simulink model "testsim_1"  (R2017b)
settings: Solver=VariableStepAuto  StartTime=0.0  StopTime=10.0  RelTol=1e-3
undefined symbols (not defined in the file or in its folder): a1, a2, a3
settings Model: Creator=rishi  LastModifiedBy=rishi

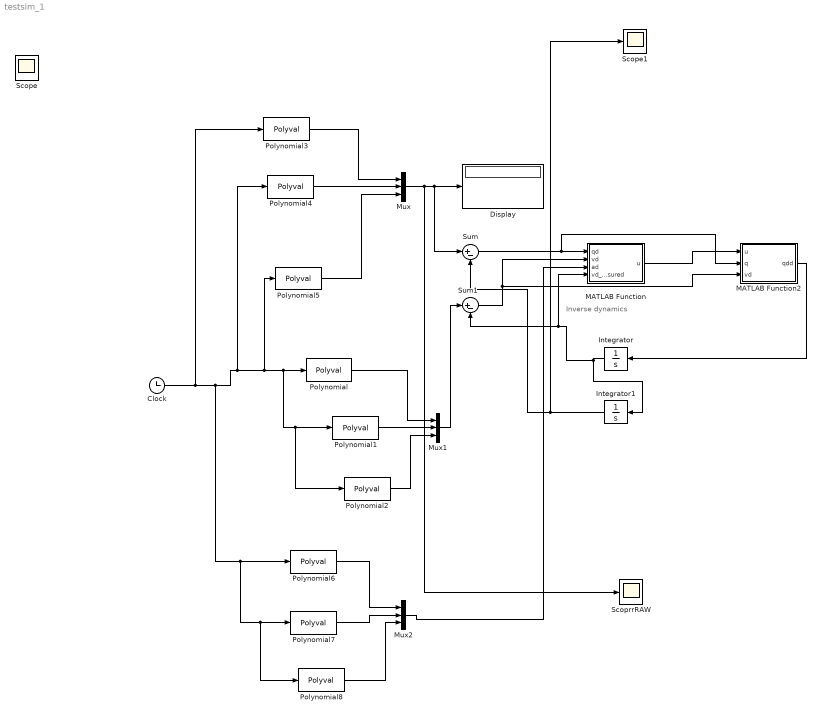
== system testsim_1 ==
  note: Inverse dynamics
  Clock : Clock
  Display : Display
  Integrator : Integrator
  Integrator1 : Integrator
  MATLAB Function : MATLAB Function  TreatAsAtomicUnit=on
  MATLAB Function2 : MATLAB Function  TreatAsAtomicUnit=on
  Mux : Mux  Inputs=3
  Mux1 : Mux  Inputs=3
  Mux2 : Mux  Inputs=3
  Polynomial : Polyval  Coefs=[a1(2) 2*a1(3) 3*a1(4)]
  Polynomial1 : Polyval  Coefs=[a2(2) 2*a2(3) 3*a2(4)]
  Polynomial2 : Polyval  Coefs=[a3(2) 2*a3(3) 3*a3(4)]
  Polynomial3 : Polyval  Coefs=[ a1(1) a1(2) a1(3) a1(4)]
  Polynomial4 : Polyval  Coefs=[ a2(1) a2(2) a2(3) a2(4)]
  Polynomial5 : Polyval  Coefs=[ a3(1) a3(2) a3(3) a3(4)]
  Polynomial6 : Polyval  Coefs=[2*a1(3) 6*a1(4)]
  Polynomial7 : Polyval  Coefs=[2*a2(3) 6*a2(4)]
  Polynomial8 : Polyval  Coefs=[2*a3(3) 6*a3(4)]
  Scope1 : Scope
  "ScoprrRAW " : Scope
  Sum : Sum  Inputs=|+-
  Sum1 : Sum  Inputs=|+-
  Scope : Scope
  wires:
  MATLAB Function2/1(qdd) -> Integrator/1
  Sum/1 -> MATLAB Function2/2(q), MATLAB Function/1(qd)
  MATLAB Function/1(u) -> MATLAB Function2/1(u)
  Sum1/1 -> MATLAB Function2/3(vd), MATLAB Function/2(vd)
  Integrator1/1 -> Scope1/1, Sum/2
  Integrator/1 -> MATLAB Function/4(vd_measured), Sum1/2, Integrator1/1
  Clock/1 -> Polynomial3/1, Polynomial8/1, Polynomial7/1, Polynomial6/1, Polynomial4/1, Polynomial5/1, Polynomial2/1, Polynomial1/1, Polynomial/1
  Mux2/1 -> MATLAB Function/3(ad)
  Polynomial/1 -> Mux1/1
  Polynomial1/1 -> Mux1/2
  Polynomial2/1 -> Mux1/3
  Polynomial6/1 -> Mux2/1
  Polynomial7/1 -> Mux2/2
  Polynomial8/1 -> Mux2/3
  Mux1/1 -> Sum1/1
  Polynomial3/1 -> Mux/1
  Polynomial4/1 -> Mux/2
  Polynomial5/1 -> Mux/3
  Mux/1 -> "ScoprrRAW "/1, Sum/1, Display/1

== matlab function testsim_1/MATLAB Function ==
  data: qd input; u output; vd input; ad input; vd_measured input


function u = fcn(qd,vd,ad,vd_measured)
Kv = diag([0.15 0.15 0.15]);
Kp = diag([0.05 0.05 0.05]);

% Kv = diag([0.000001 0.000001 0.000001]);
% Kp = diag([0.000001 0.000001 0.000001]);
%       0 1 0;
%       0 0 1;];
% Kp =  [1 0 0;
%        0 1 0;
%        0 0 1;];
ad = transpose(ad)
% vd = transpose(vd)
% qd = transpose(qd)
aq = transpose(ad - transpose(Kv*(vd)) - transpose(Kp*(qd)))
 [M,C,G]=dynamics(qd);
%  display(vd_measured)
 u = M*aq + C*vd + G
 
function [M,C,G] = dynamics(qd)
I = [0.006757, 0.0006036, 0.0015514;
    0.001745, 0.0005596, 0.00006455;
    0.00706657, 0.0006254, 0.0015708];
m = [1.01992, 0.3519, 0.22772]; % masses of the link in kg
l = [0.25107, 0.191, 0.37843];% lengths of links in m
r = [0.10424, 0.14550, 0.203];

t1= qd(1);
t2= qd(2);
t3= qd(3);

M11 = I(5)*(sin(t2)^2) + I(6)*(cos(t2+t3)^2)+ m(2)*I(7)*(cos(t2)^2)*(r(2)^2)+ m(3)*(l(1)*cos(t2)+ r(2)*cos(t2+t3))^2;
M12 = 0;
M13 = 0;
M21 = 0;

M22 = I(2) + I(3) + m(2)*(l(1))^2 + m(2)*(r(1))^2 + m(3)*(r(3))^2 +2 * m(3)*l(1)*r(2)* cos(t3);


M23 = I(3) + m(3)*(r(2))^2 + m(3)*l(1)*r(1)*cos(t3);


M31 = 0;
M32 = I(3) + m(3)*(r(1))^2 + m(3)*l(1)*r(2)*cos(t3);
M33 = I(3) + m(3)* (r(2))^2;


M =  [ M11 M12 M13;
       M21 M22 M23;
       M31 M32 M33];
%% Gravity is a bitch
g = 9.81;

G1 = 0;


G2 = -(m(2)*r(1) + m(3)*l(1))*g* cos(t2)- m(3)*r(2)*cos(t2 + t3);

G3 = -m(3)*g*r(2)*cos(t2 + t3);

G = [G1;G2;G3];
%% coriolis matrix
t23 = t2 + t3;
C = zeros(3);

gamma_001 = 0.5*( I(8) - I(9) - m(2)*r(2)^2)*sin(2*t2) + 0.5*( I(5)-I(9) )*sin(2*t23)-m(3)*(l(2)*cos(t2) + r(3)*cos(t23))*(l(2)*sin(t2) + r(3)*sin(t23));

gamma_002 = 0.5*(I(6) - I(9))*cos(2*t23) -m(3)*r(3)*sin(t23)*(l(2)*cos(t2) + r(3)*cos(t23));

gamma_010 = 0.5*(I(5) - I(8) - m(2)*r(2)^2)*cos(2*t2) + 0.5*( I(6) - I(9))*cos(2*t2)-m(3)*(l(2)*cos(t2) + r(3)*cos(t23))*(l(2)*sin(t2) + r(3)*sin(t23));


gamma_020 = 0.5*(I(6) - I(9))*sin(2*t23) -m(3)*r(3)*sin(t23)*(l(2)*cos(t2) + r(3)*cos(t23));

gamma_100 = 0.5*(I(8) - I(5) + m(2)*r(2)^2)*sin(2*t2) + 0.5*(I(9) - I(6))*sin(2*t23) + m(3)*( l(2)*cos(t2) + r(3)*cos(t23))*(l(2)*sin(t2) + r(3)*sin(t23));

gamma_112 = -l(2)*m(3)*r(2)*sin(t3);

gamma_121 = gamma_112;
gamma_122 = gamma_112;


gamma_200 = 0.5*(I(9) - I(6)) + m(2)*r(3)*sin(t23)*(l(2)*cos(t2) + r(3)*cos(t23));
gamma_211 = l(2)*m(3)*r(3)*sin(t3);


C(1) = gamma_001 + gamma_002;
C(4) = gamma_010;
C(7) = gamma_020;
C(2) = gamma_100;
C(5) = gamma_112;
C(8) = gamma_121 + gamma_122;

C(3) = gamma_200;
C(6) = gamma_211;


% qdd =  inv(M)*(u - C - G);
end    
end

== matlab function testsim_1/MATLAB Function2 ==
  data: u input; qdd output; q input; vd input

function qdd   = dynamics(u,q,vd)
I = [0.006757, 0.0006036, 0.0015514;
    0.001745, 0.0005596, 0.00006455;
    0.00706657, 0.0006254, 0.0015708];
m = [1.01992, 0.3519, 0.22772]; % masses of the link in kg
l = [0.25107, 0.191, 0.37843];% lengths of links in m
r = [0.10424, 0.14550, 0.203];
% q = [10,15,90];
t1= q(1);
t2= q(2);
t3= q(3);

M11 = I(5)*(sin(t2)^2) + I(6)*(cos(t2+t3)^2)+ m(2)*I(7)*(cos(t2)^2)*(r(2)^2)+ m(3)*(l(1)*cos(t2)+ r(2)*cos(t2+t3))^2;
M12 = 0;
M13 = 0;
M21 = 0;

M22 = I(2) + I(3) + m(2)*(l(1))^2 + m(2)*(r(1))^2 + m(3)*(r(3))^2 +2 * m(3)*l(1)*r(2)* cos(t3);


M23 = I(3) + m(3)*(r(2))^2 + m(3)*l(1)*r(1)*cos(t3);


M31 = 0;
M32 = I(3) + m(3)*(r(1))^2 + m(3)*l(1)*r(2)*cos(t3);
M33 = I(3) + m(3)* (r(2))^2;


M =  [ M11 M12 M13;
       M21 M22 M23;
       M31 M32 M33];
%% Gravity is a bitch
g = 9.81;

G1 = 0;


G2 = -(m(2)*r(1) + m(3)*l(1))*g* cos(t2)- m(3)*r(2)*cos(t2 + t3);

G3 = -m(3)*g*r(2)*cos(t2 + t3);

G = [G1;G2;G3];
%% coriolis matrix
t23 = t2 + t3;
C = zeros(3);

gamma_001 = 0.5*( I(8) - I(9) - m(2)*r(2)^2)*sin(2*t2) + 0.5*( I(5)-I(9) )*sin(2*t23)-m(3)*(l(2)*cos(t2) + r(3)*cos(t23))*(l(2)*sin(t2) + r(3)*sin(t23));

gamma_002 = 0.5*(I(6) - I(9))*cos(2*t23) -m(3)*r(3)*sin(t23)*(l(2)*cos(t2) + r(3)*cos(t23));

gamma_010 = 0.5*(I(5) - I(8) - m(2)*r(2)^2)*cos(2*t2) + 0.5*( I(6) - I(9))*cos(2*t2)-m(3)*(l(2)*cos(t2) + r(3)*cos(t23))*(l(2)*sin(t2) + r(3)*sin(t23));


gamma_020 = 0.5*(I(6) - I(9))*sin(2*t23) -m(3)*r(3)*sin(t23)*(l(2)*cos(t2) + r(3)*cos(t23));

gamma_100 = 0.5*(I(8) - I(5) + m(2)*r(2)^2)*sin(2*t2) + 0.5*(I(9) - I(6))*sin(2*t23) + m(3)*( l(2)*cos(t2) + r(3)*cos(t23))*(l(2)*sin(t2) + r(3)*sin(t23));

gamma_112 = -l(2)*m(3)*r(2)*sin(t3);

gamma_121 = gamma_112;
gamma_122 = gamma_112;


gamma_200 = 0.5*(I(9) - I(6)) + m(2)*r(3)*sin(t23)*(l(2)*cos(t2) + r(3)*cos(t23));
gamma_211 = l(2)*m(3)*r(3)*sin(t3);


C(1) = gamma_001 + gamma_002;
C(4) = gamma_010;
C(7) = gamma_020;
C(2) = gamma_100;
C(5) = gamma_112;
C(8) = gamma_121 + gamma_122;

C(3) = gamma_200;
C(6) = gamma_211;




qdd =  inv(M)*(u - C*vd - G);
end
